simulink model "planar3dof_sim"  (R2017a)
settings: Solver=ode45  StartTime=0.0  StopTime=4  MaxStep=1e-2  RelTol=1e-3  EnableMultiTasking=on
values from neighbouring files (symbols this model uses):
  K = 1    [ex3.m]    (also in mdl_kinovagen3.m = 8.91; planar3dof.m = 50)
  q0 = [-pi/20 -pi/2]'    [ex3.m]    (also in planar3dof.m = [pi -pi/2 -pi/2])
libraries: dspmtrx3 x5, roblocks x4
settings Model: Creator=alexfneves  LastModifiedBy=rbp
settings DataIOCC: LimitDataPoints=on  SaveFormat=Array
settings OptimizationCC: LifeSpan=inf
settings DebuggingCC: SFUnexpectedBacktrackingDiag=warning  SFNoUnconditionalDefaultTransitionDiag=warning  SFExecutionAtInitializationDiag=none
settings HardwareCC: ProdBitPerPointer=32  ProdBitPerSizeT=32  ProdBitPerPtrDiffT=32  ProdLargestAtomicFloat=None  ProdIntDivRoundTo=Undefined  ProdEndianess=Unspecified  ProdWordSize=32  ProdHWDeviceType=32-bit Generic
settings ModelReferenceCC: PropagateSignalLabelsOutOfModel=off
settings GRTTargetCC: TargetLangStandard=C89/C90 (ANSI)  GeneratePreprocessorConditionals=Disable all
settings ConfigComp: CovMetricSettings=dw  CovHtmlReporting=on  CovSaveCumulativeToWorkspaceVar=on  CovSaveSingleToWorkspaceVar=on  CovExternalEMLEnable=off

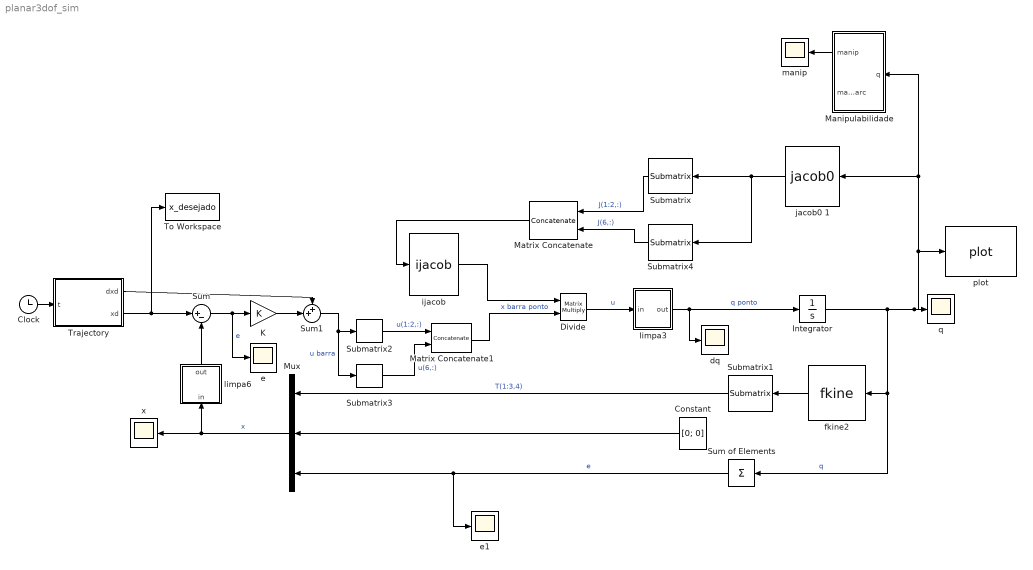
== system planar3dof_sim ==
  Clock : Clock
  Constant : Constant  Value=[0; 0]  VectorParams1D=off
  Divide : Product  Inputs=**  Multiplication=Matrix(*)
  Integrator : Integrator  InitialCondition=q0
  K : Gain  Gain=K
  Manipulabilidade : MATLAB Function  TreatAsAtomicUnit=on
  Matrix Concatenate : Concatenate  Mode=Multidimensional array
  Matrix Concatenate1 : Concatenate  Mode=Multidimensional array
  Mux : Mux  Inputs=3
  Submatrix : dspmtrx3/Submatrix  RowSpan=Range of rows  RowStartMode=First  RowStartIndex=1  RowEndMode=Index  RowEndIndex=2  ColSpan=All columns  ColStartMode=First  ColStartIndex=1  ColEndMode=Index  ColEndIndex=3
  Submatrix1 : dspmtrx3/Submatrix  RowSpan=Range of rows  RowStartMode=First  RowStartIndex=1  RowEndMode=Offset from last  RowEndIndex=1  ColSpan=One column  ColStartMode=Last  ColStartIndex=1  ColEndMode=Last  ColEndIndex=1
  Submatrix2 : dspmtrx3/Submatrix  RowSpan=Range of rows  RowStartMode=First  RowStartIndex=1  RowEndMode=Index  RowEndIndex=2  ColSpan=All columns  ColStartMode=First  ColStartIndex=1  ColEndMode=Index  ColEndIndex=3
  Submatrix3 : dspmtrx3/Submatrix  RowSpan=One row  RowStartMode=Last  RowStartIndex=1  RowEndMode=Index  RowEndIndex=2  ColSpan=All columns  ColStartMode=First  ColStartIndex=1  ColEndMode=Index  ColEndIndex=3
  Submatrix4 : dspmtrx3/Submatrix  RowSpan=One row  RowStartMode=Last  RowStartIndex=1  RowEndMode=Index  RowEndIndex=2  ColSpan=All columns  ColStartMode=First  ColStartIndex=1  ColEndMode=Index  ColEndIndex=3
  Sum : Sum  Inputs=|+-
  Sum of Elements : Sum  Inputs=+
  Sum1 : Sum  Inputs=++|
  To Workspace : ToWorkspace  VariableName=x_desejado  SaveFormat=Timeseries  SampleTime=-1
  Trajectory : MATLAB Function  TreatAsAtomicUnit=on
  dq : Scope
  e : Scope
  e1 : Scope
  fkine2 : roblocks/Arm/fkine  robot=planar
  ijacob : roblocks/Arm/ijacob
  jacob0 1 : roblocks/Arm/jacob0   robot=planar
  limpa3 : MATLAB Function  TreatAsAtomicUnit=on
  limpa6 : MATLAB Function  TreatAsAtomicUnit=on
  manip : Scope
  plot : roblocks/Arm/plot  robot=planar  fps=5  holdplot=on
  q : Scope
  x : Scope
  wires:
  Integrator/1 -> plot/1, Manipulabilidade/1(q), jacob0 1/1, q/1, fkine2/1, Sum of Elements/1  "q"
  Sum/1 -> e/1, K/1  "e"
  Clock/1 -> Trajectory/1(t)
  fkine2/1 -> Submatrix1/1
  Mux/1 -> limpa6/1(in), x/1  "x"
  Trajectory/2(xd) -> To Workspace/1, Sum/1
  K/1 -> Sum1/2
  Trajectory/1(dxd) -> Sum1/1
  Submatrix1/1 -> Mux/1  "T(1:3,4)"
  Constant/1 -> Mux/2
  Divide/1 -> limpa3/1(in)  "u"
  Submatrix2/1 -> Matrix Concatenate1/1  "u(1:2,:)"
  Submatrix3/1 -> Matrix Concatenate1/2  "u(6,:)"
  Sum1/1 -> Submatrix3/1, Submatrix2/1  "u barra"
  Matrix Concatenate1/1 -> Divide/2  "x barra ponto"
  Submatrix4/1 -> Matrix Concatenate/2  "J(6,:)"
  Submatrix/1 -> Matrix Concatenate/1  "J(1:2,:)"
  jacob0 1/1 -> Submatrix/1, Submatrix4/1
  Matrix Concatenate/1 -> ijacob/1
  ijacob/1 -> Divide/1
  limpa6/1(out) -> Sum/2
  limpa3/1(out) -> dq/1, Integrator/1  "q ponto"
  Sum of Elements/1 -> e1/1, Mux/3  "e"
  Manipulabilidade/1(manip) -> manip/1

== matlab function planar3dof_sim/limpa6 ==
  data: out output; in input
function out = limpa(in)
%#codegen
    out = [in(1) in(2) in(3) in(4) in(5) in(6)]'
end

== matlab function planar3dof_sim/Trajectory ==
  data: dxd output; xd output; t input
function [dxd, xd] = trajectory(t)
%#codegen

    xd = xdFunc(t);
    dxd = dxdFunc(t);
end

== matlab function planar3dof_sim/limpa3 ==
  data: out output; in input
function out = limpa(in)
%#codegen
    out = [in(1) in(2) in(3)]'
end

== matlab function planar3dof_sim/Manipulabilidade ==
  data: q input; manip output; manip_parc output
function [manip, manip_parc] = Manip(q)
%#codegen

[manip, manip_parc] = manipFunc(q(1), q(2), q(3));
